simulink subsystem "Sensor_Input_Block_ThorneFleissner"  (R2020b)
settings: Solver=VariableStepAuto  StartTime=0.0  StopTime=10.0  RelTol=1e-3
settings Model: Creator=rthom  LastModifiedBy=rthom

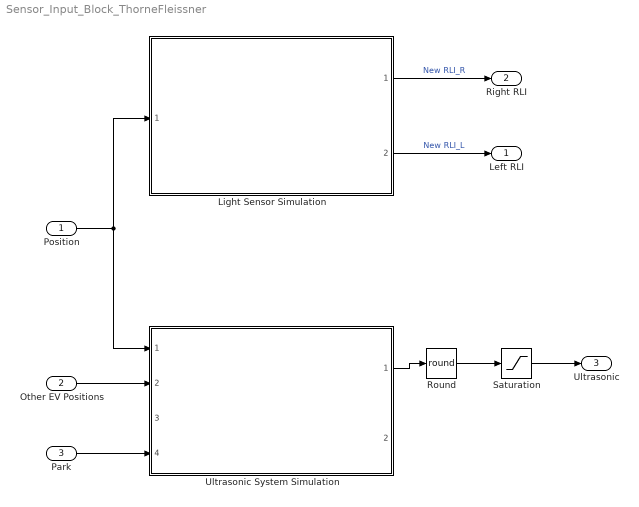
== system Sensor_Input_Block_ThorneFleissner ==
  Position : Inport
  Other EV Positions : Inport  Port=2
  Park : Inport  Port=3
  Light Sensor Simulation : Subsystem  ReferencedSubsystem=Light_Sensor_Simulation_ThorneFleissner
  Round : Rounding  Operator=round
  Saturation : Saturate  UpperLimit=255  LowerLimit=0
  Ultrasonic System Simulation : Subsystem  ReferencedSubsystem=Ultrasonic_System_Simulation_ThorneFleissner
  Left RLI : Outport
  Right RLI : Outport  Port=2
  Ultrasonic : Outport  Port=3
  wires:
  Position/1 -> Ultrasonic System Simulation/1, Light Sensor Simulation/1
  Light Sensor Simulation/1 -> Right RLI/1  "New RLI_R"
  Light Sensor Simulation/2 -> Left RLI/1  "New RLI_L"
  Ultrasonic System Simulation/1 -> Round/1
  Park/1 -> Ultrasonic System Simulation/4
  Other EV Positions/1 -> Ultrasonic System Simulation/2
  Round/1 -> Saturation/1
  Saturation/1 -> Ultrasonic/1
